simulink model "Engine_TestModel"  (R2025a)
settings: Solver=ode23t  StartTime=0.0  StopTime=10.0  RelTol=1e-3
undefined symbols (not defined in the file or in its folder): GroundAmbientTemp_K
libraries: nesl_utility x5, SimscapeFluids_lib x4, fl_lib x3, simulink x1
settings Model: Creator=Adam  LastModifiedBy=Adam
settings DataIOCC: InspectSignalLogs=on
settings SimscapeCC: SimscapeLogType=all  SimscapeLogSimulationStatistics=on  SimscapeLogToSDI=on

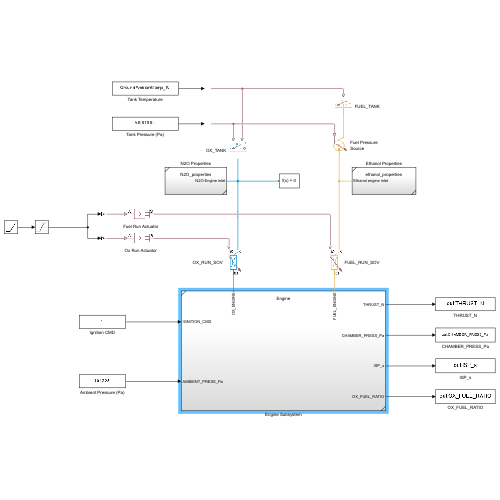
[thumbnail: Simulink's stored preview of the top-level diagram]
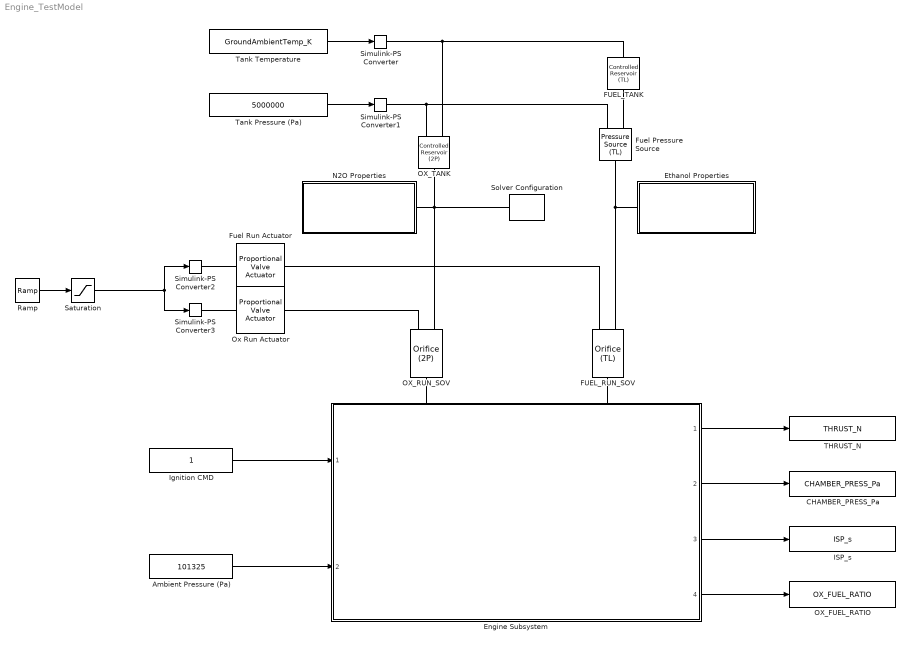
== system Engine_TestModel ==
  Ambient Pressure (Pa) : Constant  Value=101325
  CHAMBER_PRESS_Pa : ToWorkspace  VariableName=CHAMBER_PRESS_Pa  SaveFormat=Timeseries  SampleTime=-1
  Engine Subsystem : Subsystem  ReferencedSubsystem=Engine
      settings: PortSchema="{\"entries\":[{\"content\":{\"sides\":[{\"content\":{\"connectorIds\":[\"In1\",\"In2\"]},\"type\":\"ConnectorPlacement.EquallySpacedRectSide\",\"uuid\":\"b0db93f8-a7dd-49b2-aa84-f89f4af0da0d\"},{\"content\":{\"connectorIds\":[\"Out1\",\"Out2\",\"Out3\",\"Out4\"],\"side\":\"RIGHT\"},\"type\":\"ConnectorPlacement.EquallySpacedRectSide\",\"uuid\":\"4ee3e158-77d6-4983-9bcd-9da779590486\"},{\"content\":{\"connectorIds\":[\"LConn1\",\"LConn2\"],\"side\":\"TOP\"},\"type\":\"ConnectorPlacement.EquallySpacedRectSide\",\"uuid\":\"9bbcc461-3fab-44f8-8c41-c071f9f93a71\"}]},\"type\":\"ConnectorPlacement.EquallySpacedConnector\",\"uuid\":\"5ac2f051-1f6f-4951-a2a3-cc1c3801f20a\"}],\"packageUris\":[\"http://schema.mathworks.com/mf0/Connector/R2020b\"],\"version\":\"1.0\"}"
  Ethanol Properties : Subsystem  ReferencedSubsystem=ethanol_properties
  FUEL_RUN_SOV : SimscapeFluids_lib/Thermal Liquid/Valves & Orifices/Orifice (TL)  orifice_type=foundation.enum.constant_variable.variable  constant_orifice_spec=fluids.thermal_liquid.valves.enum.ConstantOrificeSpec.Area  variable_orifice_spec=fluids.thermal_liquid.valves.enum.orifice_spec.linear  orifice_area_constant=1e-3 m^2  p_diff_TLU_constant=[-4, -3, -2, -1, -.5, 0, .5, 1, 2, 3, 4] MPa  vol_flow_TLU_constant=[-2.44, -2.12, -1.68, -1.22, -.84, 0, .85, 1.21, 1.7, 2.09, 2.41] .* 1e-3 m^3/s  mdot_TLU_constant=[-2.44, -2.12, -1.68, -1.22, -.84, 0, .85, 1.21, 1.7, 2.09, 2.41] kg/s  S_min=0 m  del_S=5e-3 m  open_orientation=fluids.thermal_liquid.valves.enum.orifice_orientation.positive  area_max=1e-4 m^2  area_leak=1e-10 m^2  S_TLU=[0, .002, .004, .007, .017] m  orifice_area_TLU=[1e-09, 2.0352e-07, 4.0736e-05, .00011438, .00034356] m^2  Cd=0.64  Re_c=150  smoothing_factor=0.01  pressure_recovery=false  S_flow_TLU=[0, .002, .004, .007, .017] m  p_diff_TLU=[.3, .5, .7] MPa  vol_flow_TLU=1e-3 * [1.7e-05, 2e-05, 2.6e-05; .0035, .0045, .0053; .7, .9, 1.06; 1.96, 2.5, 3; 6, 7.7, 9.13] m^3/s  mdot_TLU=[1.7e-05, 2e-05, 2.6e-05; .0035, .0045, .0053; .7, .9, 1.06; 1.96, 2.5, 3; 6, 7.7, 9.13] kg/s  T_ref_in=293.15 K  p_ref_in=0.101325 MPa  area=0.01 m^2
      settings: InternalSimscapePortConfiguration="{\"Bottom\":[],\"Left\":[{\"id\":\"A\",\"label\":\"A\",\"type\":\"foundation.thermal_liquid.thermal_liquid\"},{\"id\":\"S\",\"label\":\"S\",\"type\":\"input\"}],\"Right\":[{\"id\":\"B\",\"label\":\"B\",\"type\":\"foundation.thermal_liquid.thermal_liquid\"}],\"Top\":[]}"
  FUEL_TANK : fl_lib/Thermal Liquid/Elements/Controlled Reservoir (TL)  pressure_spec=foundation.enum.pressure_spec.atmospheric  reservoir_pressure=0.101325 MPa  area=0.01 m^2
      settings: InternalSimscapePortConfiguration="{\"Bottom\":[],\"Left\":[{\"id\":\"A\",\"label\":\"A\",\"type\":\"foundation.thermal_liquid.thermal_liquid\"}],\"Right\":[{\"id\":\"T_in\",\"label\":\"T\",\"type\":\"input\"}],\"Top\":[]}"
  Fuel Pressure Source : fl_lib/Thermal Liquid/Sources/Pressure Source (TL)  source_type=foundation.enum.constant_controlled.controlled  pressure_differential=0 MPa  power_spec=foundation.enum.power_spec.isentropic  area=0.01 m^2
      settings: InternalSimscapePortConfiguration="{\"Bottom\":[],\"Left\":[{\"id\":\"A\",\"label\":\"A\",\"type\":\"foundation.thermal_liquid.thermal_liquid\"},{\"id\":\"P\",\"label\":\"P\",\"type\":\"input\"}],\"Right\":[{\"id\":\"B\",\"label\":\"B\",\"type\":\"foundation.thermal_liquid.thermal_liquid\"}],\"Top\":[]}"
  Fuel Run Actuator : SimscapeFluids_lib/Valve Actuators/Proportional Valve Actuator  gain=5e-3 m  time_constant=0.01 s  valve_stroke=0.005 m
      settings: InternalSimscapePortConfiguration="{\"Bottom\":[],\"Left\":[{\"id\":\"A\",\"label\":\"A\",\"type\":\"input\"}],\"Right\":[{\"id\":\"S\",\"label\":\"S\",\"type\":\"output\"}],\"Top\":[]}"
  ISP_s : ToWorkspace  VariableName=ISP_s  SaveFormat=Timeseries  SampleTime=-1
  Ignition CMD : Constant
  N2O Properties : Subsystem  ReferencedSubsystem=N2O_properties
  OX_FUEL_RATIO : ToWorkspace  VariableName=OX_FUEL_RATIO  SaveFormat=Timeseries  SampleTime=-1
  OX_RUN_SOV : SimscapeFluids_lib/Two-Phase Fluid/Valves & Orifices/Orifice (2P)  orifice_type=foundation.enum.constant_variable.variable  constant_liquid_orifice_parameterization=fluids.two_phase_fluid.valves_orifices.enum.LiquidConstantOrificeParameterization.Area  variable_liquid_orifice_parameterization=fluids.two_phase_fluid.valves_orifices.enum.LiquidOrificeParameterization.LinearArea  mdot_nominal_constant=0.1 kg/s  delta_p_nominal_constant=0.001 MPa  orifice_area_constant=1e-4 m^2  S_min=0 m  del_S=5e-3 m  open_orientation=fluids.two_phase_fluid.valves_orifices.enum.OrificeOrientation.Positive  mdot_nominal_max=0.1 kg/s  delta_p_nominal_max=0.001 MPa  orifice_area_max=1e-4 m^2  S_TLU=[0, .002, .004, .007, .017] m  orifice_area_TLU=[1e-10, 2e-05, 4e-05, 6e-05, 8e-05, .0001] m^2  energy_spec=foundation.enum.energy_spec.temperature  p_inlet=0.101325 MPa  T_inlet=293.15 K  x_inlet=0  alpha_inlet=0  h_inlet=400 kJ/kg  u_inlet=400 kJ/kg  Cd=0.64  pressure_recovery=false  leakage_fraction=1e-6  smoothing_factor=0.01  B_lam=0.999  tau_x=0.1 s  area=0.01 m^2  vapor_orifice_parameterization=fluids.two_phase_fluid.valves_orifices.enum.VaporOrificeParameterization.Cv  opening_characteristic=fluids.two_phase_fluid.valves_orifices.enum.OpeningCharacteristics.Linear  Cv_constant=4  Cv_max=4  S_Cv_TLU=[0, .003, .006, .009, .012, .015] m  Cv_TLU=[1e-06, .8, 1.6, 2.4, 3.2, 4]  xT_Cv=0.7  Kv_constant=3.6  Kv_max=3.6  S_Kv_TLU=[0, .003, .006, .009, .012, .015] m  Kv_TLU=[1e-06, .72, 1.44, 2.16, 2.88, 3.6]  xT_Kv=0.7  S_orifice_area_TLU=[0, .003, .006, .009, .012, .015] m
      settings: InternalSimscapePortConfiguration="{\"Bottom\":[],\"Left\":[{\"id\":\"A\",\"label\":\"A\",\"type\":\"foundation.two_phase_fluid.two_phase_fluid\"},{\"id\":\"S\",\"label\":\"S\",\"type\":\"input\"}],\"Right\":[{\"id\":\"B\",\"label\":\"B\",\"type\":\"foundation.two_phase_fluid.two_phase_fluid\"}],\"Top\":[]}"
  OX_TANK : fl_lib/Two-Phase Fluid/Elements/Controlled Reservoir (2P)  pressure_spec=foundation.enum.ControlledReservoirPressureSpec2P.Specified  energy_spec=foundation.enum.ControlledReservoirEnergySpec2P.LiquidTemperature  area_A=0.01 m^2  pressure_limit_spec=foundation.enum.PressureLimitSpec2P.Warn
      settings: InternalSimscapePortConfiguration="{\"Bottom\":[],\"Left\":[{\"id\":\"A\",\"label\":\"A\",\"type\":\"foundation.two_phase_fluid.two_phase_fluid\"}],\"Right\":[{\"id\":\"T\",\"label\":\"T\",\"type\":\"input\"},{\"id\":\"P\",\"label\":\"P\",\"type\":\"input\"}],\"Top\":[]}"
  Ox Run Actuator : SimscapeFluids_lib/Valve Actuators/Proportional Valve Actuator  gain=5e-3 m  time_constant=0.01 s  valve_stroke=0.005 m
      settings: InternalSimscapePortConfiguration="{\"Bottom\":[],\"Left\":[{\"id\":\"A\",\"label\":\"A\",\"type\":\"input\"}],\"Right\":[{\"id\":\"S\",\"label\":\"S\",\"type\":\"output\"}],\"Top\":[]}"
  Ramp : simulink/Sources/Ramp  slope=1  start=3  InitialOutput=0
  Saturation : Saturate  UpperLimit=1  LowerLimit=0
  Simulink-PS Converter : nesl_utility/Simulink-PS Converter  PhysicalDomain=network_engine_domain  SubClassName=ps_input  LeftPortType=input  RightPortType=output  PseudoPeriodic=off  Frequencies=[]  NoiseDistribution=none  NoiseParameters=[]  Unit=K  AffineConversion=off  FilteringAndDerivatives=provide  SimscapeFilterOrder=1  InputFilterTimeConstant=0.001  UdotUserProvided=0
  Simulink-PS Converter1 : nesl_utility/Simulink-PS Converter  PhysicalDomain=network_engine_domain  SubClassName=ps_input  LeftPortType=input  RightPortType=output  PseudoPeriodic=off  Frequencies=[]  NoiseDistribution=none  NoiseParameters=[]  Unit=Pa  AffineConversion=off  FilteringAndDerivatives=provide  SimscapeFilterOrder=1  InputFilterTimeConstant=0.001  UdotUserProvided=0
  Simulink-PS Converter2 : nesl_utility/Simulink-PS Converter  PhysicalDomain=network_engine_domain  SubClassName=ps_input  LeftPortType=input  RightPortType=output  PseudoPeriodic=off  Frequencies=[]  NoiseDistribution=none  NoiseParameters=[]  Unit=K  AffineConversion=off  FilteringAndDerivatives=provide  SimscapeFilterOrder=1  InputFilterTimeConstant=0.001  UdotUserProvided=0
  Simulink-PS Converter3 : nesl_utility/Simulink-PS Converter  PhysicalDomain=network_engine_domain  SubClassName=ps_input  LeftPortType=input  RightPortType=output  PseudoPeriodic=off  Frequencies=[]  NoiseDistribution=none  NoiseParameters=[]  Unit=K  AffineConversion=off  FilteringAndDerivatives=provide  SimscapeFilterOrder=1  InputFilterTimeConstant=0.001  UdotUserProvided=0
  Solver Configuration : nesl_utility/Solver Configuration  PhysicalDomain=network_engine_domain  SubClassName=solver  LeftPortType=input  RightPortType=generic  Tones=[]  Harmonics=[]  SimulateNoise=off  Profile=off  UseLocalSampling=off  EnableSwitchedLinearOptims=on  FrequencyDomain=off  UseCCode=off  RelTol=0.001  AbsTol=0.001  MinStep=1e-09  ToWorkspace=off  RevertToSquareIcSolve=off  NumHomotopyIterations=100  PhasorMode=off  PhasorModeNumHarmonics=1  ConsistencySolver=NEWTON_XTOL_AFTER_FTOL  IndexReductionMethod=DerivativeReplacement  DoDC=off  ResidualTolerance=1e-09  ConsistencyTolSource=GLOBAL  ConsistencyAbsTol=0.001  ConsistencyRelTol=0.001  ConsistencyTolFactor=0.001  UseLocalSolver=off  LocalSolverChoice=NE_BACKWARD_EULER_ADVANCER  ResolveIndetEquations=on  FunctionEvalNumThread=1  LocalSolverSampleTime=0.001  DoFixedCost=off  MaxNonlinIter=3  MaxModeIter=2  ComputeImpulses=off  ImpulseIterations=2  LinearAlgebra=auto  LinearAlgebraNumThread=0  EquationFormulation=NE_TIME_EF  DelaysMemoryBudget=1024  AutomaticFiltering=on  FilteringTimeConstant=0.001  PartitionStorageMethod=AS_NEEDED  PartitionMemoryBudget=1024  PartitionMethod=ROBUST  MultibodyUseLocalSolver=off  MultibodyLocalSolverChoice=ODE1  MultibodyLocalSolverSampleTime=0.001
  THRUST_N : ToWorkspace  VariableName=THRUST_N  SaveFormat=Timeseries  SampleTime=-1
  Tank Pressure (Pa) : Constant  Value=5000000
  Tank Temperature : Constant  Value=GroundAmbientTemp_K
  wires:
  Tank Temperature/1 -> Simulink-PS Converter/1
  Tank Pressure (Pa)/1 -> Simulink-PS Converter1/1
  Ignition CMD/1 -> Engine Subsystem/1
  Engine Subsystem/1 -> THRUST_N/1
  Engine Subsystem/2 -> CHAMBER_PRESS_Pa/1
  Ambient Pressure (Pa)/1 -> Engine Subsystem/2
  Engine Subsystem/3 -> ISP_s/1
  Engine Subsystem/4 -> OX_FUEL_RATIO/1
  Saturation/1 -> Simulink-PS Converter2/1, Simulink-PS Converter3/1
  Ramp/1 -> Saturation/1
  connections:
  Ethanol Properties/LConn1 -- Fuel Pressure Source/RConn1 -- FUEL_RUN_SOV/LConn1
  N2O Properties/LConn1 -- Solver Configuration/RConn1 -- OX_RUN_SOV/LConn1 -- OX_TANK/LConn1
  OX_TANK/RConn1 -- Simulink-PS Converter/RConn1 -- FUEL_TANK/RConn1
  Simulink-PS Converter1/RConn1 -- OX_TANK/RConn2 -- Fuel Pressure Source/LConn2
  Engine Subsystem/LConn1 -- OX_RUN_SOV/RConn1
  Engine Subsystem/LConn2 -- FUEL_RUN_SOV/RConn1
  Ox Run Actuator/RConn1 -- OX_RUN_SOV/LConn2
  Fuel Run Actuator/RConn1 -- FUEL_RUN_SOV/LConn2
  Fuel Pressure Source/LConn1 -- FUEL_TANK/LConn1
  Simulink-PS Converter2/RConn1 -- Fuel Run Actuator/LConn1
  Simulink-PS Converter3/RConn1 -- Ox Run Actuator/LConn1
